simulink model "Mit_law_2"  (Simulink 7.3)
settings: Solver=ode5  StartTime=0.0  StopTime=200  FixedStep=0.01  RelTol=1e-3
StopFcn:
  | subplot(211);
  | plot(Data.time,Data.signals(1).values(:,1),'r',Data.time,Data.signals(1).values(:,2),'b')
  | subplot(212);
  | plot(Data.time,Data.signals(2).values(:,1),'b')
settings Model: Creator=Minh-Map-Vu  LastModifiedBy=nthuy
settings DataIOCC: SignalLoggingName=sigsOut
settings DebuggingCC: SaveWithParameterizedLinksMsg=none  SignalResolutionControl=TryResolveAllWithWarning  SolverPrmCheckMsg=none  MultiTaskDSMMsg=warning  MultiTaskCondExecSysMsg=none  StrictBusMsg=None
settings HardwareCC: TargetUnknown=on
settings RTWCC: IncludeERTFirstTime=on

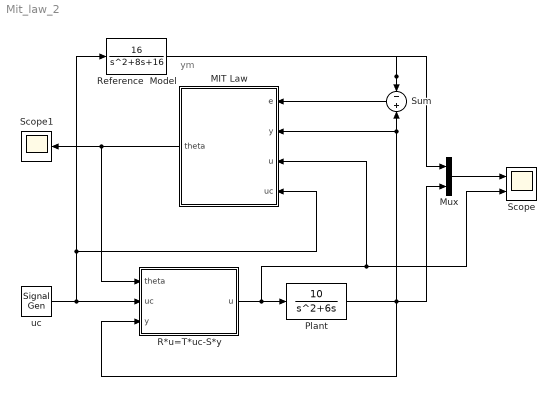
== system Mit_law_2 ==
  note: ym
  MIT Law : Subsystem
  Mux : Mux  Inputs=2
  Plant : TransferFcn  Numerator=10  Denominator="[1 6  0]"
  R*u=T*uc-S*y : Subsystem
  Reference  Model : TransferFcn  Numerator=[16]  Denominator=[1 8 16]
  Scope : Scope  NumInputPorts=2
      settings: TimeRange=100  YMin=-1.2~-5  YMax=1.2~5  SaveName=Data
  Scope1 : Scope
      settings: TimeRange=100  YMin=0  YMax=30  SaveName=Data1
  Sum : Sum  Inputs=-+  SaturateOnIntegerOverflow=on
  uc : SignalGenerator  WaveForm=square  Frequency=1/20
  wires:
  Mux/1 -> Scope/1
  uc/1 -> R*u=T*uc-S*y/2(uc), Reference  Model/1, MIT Law/4(uc)
  Reference  Model/1 -> Sum/1, Mux/1
  Plant/1 -> Sum/2, MIT Law/2(y), R*u=T*uc-S*y/3(y), Mux/2
  Sum/1 -> MIT Law/1(e)
  MIT Law/1(theta) -> Scope1/1, R*u=T*uc-S*y/1(theta)
  R*u=T*uc-S*y/1(u) -> Plant/1, MIT Law/3(u), Scope/2

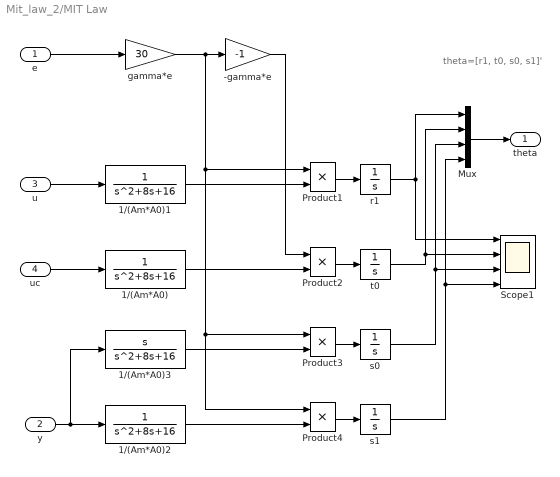
== system Mit_law_2/MIT Law ==
  note: theta=[r1, t0, s0, s1]'
  e : Inport
  y : Inport  Port=2
  u : Inport  Port=3
  uc : Inport  Port=4
  -gamma*e : Gain  Gain=-1  SaturateOnIntegerOverflow=on  OutDataTypeStr=Inherit: Same as input  ParamDataTypeStr=Inherit: Same as input
  1/(Am*A0) : TransferFcn  Numerator=1  Denominator=[1 8 16]
  1/(Am*A0)1 : TransferFcn  Numerator=1  Denominator=[1 8 16]
  1/(Am*A0)2 : TransferFcn  Numerator=1  Denominator=[1 8 16]
  1/(Am*A0)3 : TransferFcn  Numerator=[1 0]  Denominator=[1 8 16]
  Mux : Mux
  Product{1..4} (4 alike) : Product  SaturateOnIntegerOverflow=on  OutDataTypeStr=Inherit: Same as first input
  Scope1 : Scope  NumInputPorts=4
      settings: TimeRange=100  YMin=-1.1~-5~-5~-5  YMax=1.1~5~5~5  SaveName=Data2
  gamma*e : Gain  Gain=30  SaturateOnIntegerOverflow=on  OutDataTypeStr=Inherit: Same as input  ParamDataTypeStr=Inherit: Same as input
  r1 : Integrator  InitialCondition=20*rand  LimitOutput=on  LowerSaturationLimit=0
  s0 : Integrator  InitialCondition=20*rand  LimitOutput=on  LowerSaturationLimit=0
  s1 : Integrator  InitialCondition=20*rand  LimitOutput=on  LowerSaturationLimit=0
  t0 : Integrator  InitialCondition=20*rand  LimitOutput=on  LowerSaturationLimit=0
  theta : Outport
  wires:
  Mux/1 -> theta/1
  uc/1 -> 1/(Am*A0)/1
  e/1 -> gamma*e/1
  y/1 -> 1/(Am*A0)2/1, 1/(Am*A0)3/1
  u/1 -> 1/(Am*A0)1/1
  gamma*e/1 -> -gamma*e/1, Product1/1, Product4/1, Product3/1
  Product1/1 -> r1/1
  1/(Am*A0)1/1 -> Product1/2
  1/(Am*A0)/1 -> Product2/2
  Product2/1 -> t0/1
  -gamma*e/1 -> Product2/1
  Product3/1 -> s0/1
  Product4/1 -> s1/1
  1/(Am*A0)2/1 -> Product4/2
  1/(Am*A0)3/1 -> Product3/2
  r1/1 -> Mux/1, Scope1/1
  t0/1 -> Mux/2, Scope1/2
  s0/1 -> Mux/3, Scope1/3
  s1/1 -> Mux/4, Scope1/4

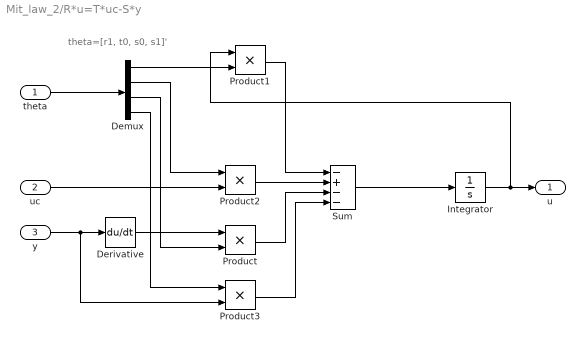
== system Mit_law_2/R*u=T*uc-S*y ==
  note: theta=[r1, t0, s0, s1]'
  theta : Inport
  uc : Inport  Port=2
  y : Inport  Port=3
  Demux : Demux
  Derivative : Derivative
  Integrator : Integrator
  Product{,1..3} (4 alike) : Product  SaturateOnIntegerOverflow=on  OutDataTypeStr=Inherit: Same as first input
  Sum : Sum  Inputs=-+--  SaturateOnIntegerOverflow=on
  u : Outport
  wires:
  Integrator/1 -> u/1, Product1/1
  y/1 -> Derivative/1, Product3/2
  Derivative/1 -> Product/1
  theta/1 -> Demux/1
  uc/1 -> Product2/2
  Product2/1 -> Sum/2
  Product1/1 -> Sum/1
  Product/1 -> Sum/3
  Product3/1 -> Sum/4
  Sum/1 -> Integrator/1
  Demux/1 -> Product1/2
  Demux/2 -> Product2/1
  Demux/3 -> Product/2
  Demux/4 -> Product3/1
